simulink model "simple_pendulum_ode"  (R2021b)
settings: Solver=ode1  StartTime=0.0  StopTime=15  FixedStep=0.001  RelTol=1e-3
settings Model: Creator=oscar  LastModifiedBy=oscar

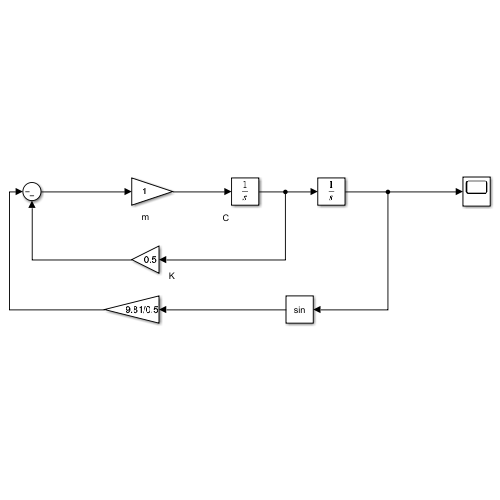
[thumbnail: Simulink's stored preview of the top-level diagram]
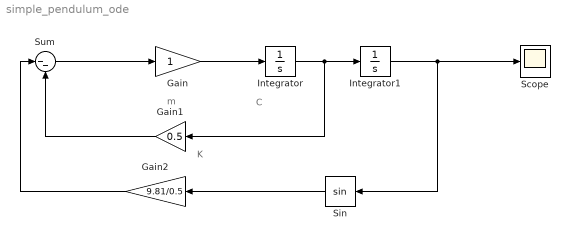
== system simple_pendulum_ode ==
  note: K
  note: m
  note: C
  Gain : Gain
  Gain1 : Gain  Gain=0.5
  Gain2 : Gain  Gain=9.81/0.5
  Integrator : Integrator
  Integrator1 : Integrator  InitialCondition=-pi/2
  Scope : Scope
  Sin : Trigonometry
  Sum : Sum  Inputs=|--
  wires:
  Gain1/1 -> Sum/2
  Gain2/1 -> Sum/1
  Gain/1 -> Integrator/1
  Integrator/1 -> Gain1/1, Integrator1/1
  Integrator1/1 -> Sin/1, Scope/1
  Sum/1 -> Gain/1
  Sin/1 -> Gain2/1
